simulink model "Not_Model"  (R2025a)
settings: Solver=VariableStepAuto  StartTime=0.0  StopTime=10.0  RelTol=1e-3
libraries: NSA_DEVS_SINKS x3, NSA_DEVS_MATH_OPERATIONS x1, NSA_DEVS_LOGISTICS x1, NSA_DEVS_SOURCES x1
settings Model: Creator=david  LastModifiedBy=peter
settings RTWCC: GPUComputeCapability=3.5

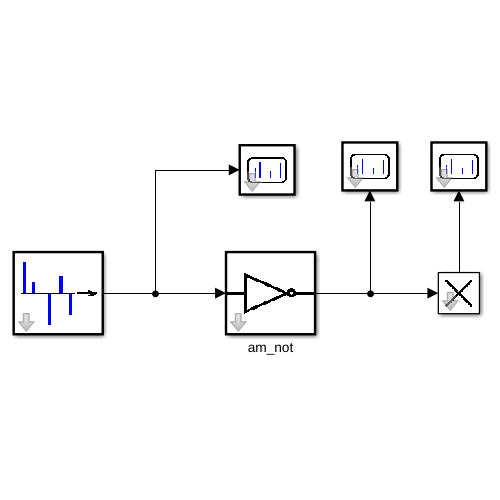
[thumbnail: Simulink's stored preview of the top-level diagram]
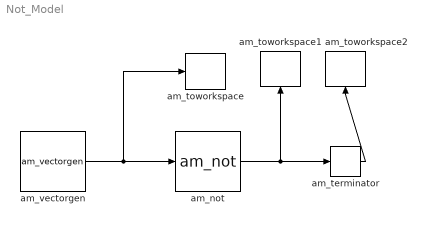
== system Not_Model ==
  am_not : NSA_DEVS_MATH_OPERATIONS/am_not  i0=true  tau_copy=[0,1]  debug_copy=0
      settings: SourceProductName=Math Operations
  am_terminator : NSA_DEVS_LOGISTICS/am_terminator  countyEmptyInputs=true  tau_copy=[0,1]  debug_copy=0
      settings: SourceProductName=Logistics
  am_toworkspace : NSA_DEVS_SINKS/am_toworkspace  varname="\"genOut\""  t0=0  format="\"vector\""  tau=[0,5]  debug=0
      settings: SourceProductName=Sinks
  am_toworkspace1 : NSA_DEVS_SINKS/am_toworkspace  varname="\"notOut\""  t0=0  format="\"vector\""  tau=[0,5]  debug=0
      settings: SourceProductName=Sinks
  am_toworkspace2 : NSA_DEVS_SINKS/am_toworkspace  varname="\"nOut\""  t0=0  format="\"vector\""  tau=[0,5]  debug=0
      settings: SourceProductName=Sinks
  am_vectorgen : NSA_DEVS_SOURCES/am_vectorgen  tvec=[0 1 2 3 4 5 6 100]  yvec=[0 1 0 1 1 0 1 0]  tau=[0,1]  debug=0
      settings: SourceProductName=Sources
  wires:
  am_vectorgen/1 -> am_not/1, am_toworkspace/1
  am_not/1 -> am_terminator/1, am_toworkspace1/1
  am_terminator/1 -> am_toworkspace2/1
